simulink model "Guidline_Fuel_Filter_Model"  (R2019a)
settings: Solver=FixedStepDiscrete  StartTime=0.0  StopTime=50  FixedStep=0.01  RelTol=1e-3
undefined symbols (not defined in the file or in its folder): Constant_0, Constant_1, Constant_100, Constant_5, Constant_50, Error_code_101, Error_code_102, resistance_constant
libraries: simulink x2
settings Model: DataDictionary=Fuel_filter_1.sldd  OrderedModelArguments=off  Creator=Akshay  LastModifiedBy=Akshay
settings OptimizationCC: DefaultParameterBehavior=Inlined  UseDivisionForNetSlopeComputation=UseDivisionForReciprocalsOfIntegersOnly  EnhancedBackFolding=on  PassReuseOutputArgsAs=Individual arguments  OptimizeBlockOrder=speed  DifferentSizesBufferReuse=on  OptimizationCustomize=off
settings DebuggingCC: SignalInfNanChecking=warning  ParameterOverflowMsg=none  ParameterTunabilityLossMsg=error  UniqueDataStoreMsg=warning  AssertControl=DisableAll  StrictBusMsg=ErrorOnBusTreatedAsVector  SFUndirectedBroadcastEventsDiag=error
settings SFSimCC: CompileTimeRecursionLimit=0  EnableRuntimeRecursion=off  MATLABDynamicMemAlloc=off
settings RTWCC: SystemTargetFile=ert.tlc  GenCodeOnly=on  TemplateMakefile=ert_default_tmf  GenerateReport=on  IncludeHyperlinkInReport=on  LaunchReport=on  GenerateTraceInfo=on  GenerateTraceReport=on  GenerateTraceReportSl=on  GenerateTraceReportSf=on  GenerateTraceReportEml=on
settings CodeAppCC: ForceParamTrailComments=on  IgnoreCustomStorageClasses=off  OperatorAnnotations=on  SimulinkDataObjDesc=on  SFDataObjDesc=on  MATLABFcnDesc=on  InsertBlockDesc=on
settings ERTTargetCC: TargetLangStandard=C99 (ISO)  UtilityFuncGeneration=Shared location  GenerateSampleERTMain=on  SupportNonFinite=off  ParenthesesLevel=Maximum  CastingMode=Standards  GenerateSharedConstants=off  InlinedParameterPlacement=NonHierarchical  ERTCustomFileTemplate=example_file_process.tlc  EnableSignedLeftShifts=off  EnableSignedRightShifts=off
settings ConfigComp: CovMetricSettings=dcmwe  DVMaxProcessTime=1000  DVParametersUseConfig=on  DVModelCoverageObjectives=MCDC  DVTestSuiteOptimization=Auto  DVDetectOutOfBounds=on  DVDetectInfNaN=on  DVDetectSubnormal=on  DVDesignMinMaxCheck=on  DVProvingStrategy=ProveWithViolationDetection  DVSaveReport=on  DVReportPDFFormat=on  DVRebuildModelRepresentation=Always

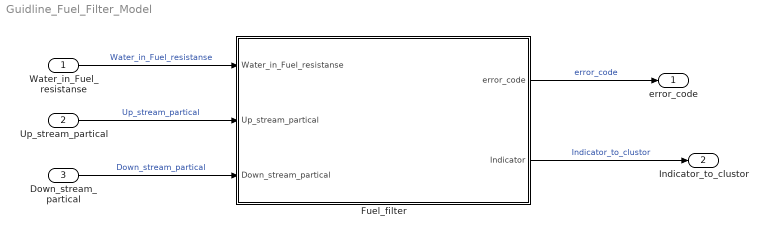
== system Guidline_Fuel_Filter_Model ==
  Water_in_Fuel_resistanse : Inport  OutDataTypeStr=single
  Up_stream_partical : Inport  Port=2  OutDataTypeStr=single
  Down_stream_partical : Inport  Port=3  OutDataTypeStr=single
  Fuel_filter : Subsystem  TreatAsAtomicUnit=on
  error_code : Outport  OutDataTypeStr=single
  Indicator_to_clustor : Outport  Port=2  OutDataTypeStr=boolean
  wires:
  Fuel_filter/1(error_code) -> error_code/1  "error_code"
  Fuel_filter/2(Indicator) -> Indicator_to_clustor/1  "Indicator_to_clustor"
  Water_in_Fuel_resistanse/1 -> Fuel_filter/1(Water_in_Fuel_resistanse)  "Water_in_Fuel_resistanse"
  Up_stream_partical/1 -> Fuel_filter/2(Up_stream_partical)  "Up_stream_partical"
  Down_stream_partical/1 -> Fuel_filter/3(Down_stream_partical)  "Down_stream_partical"

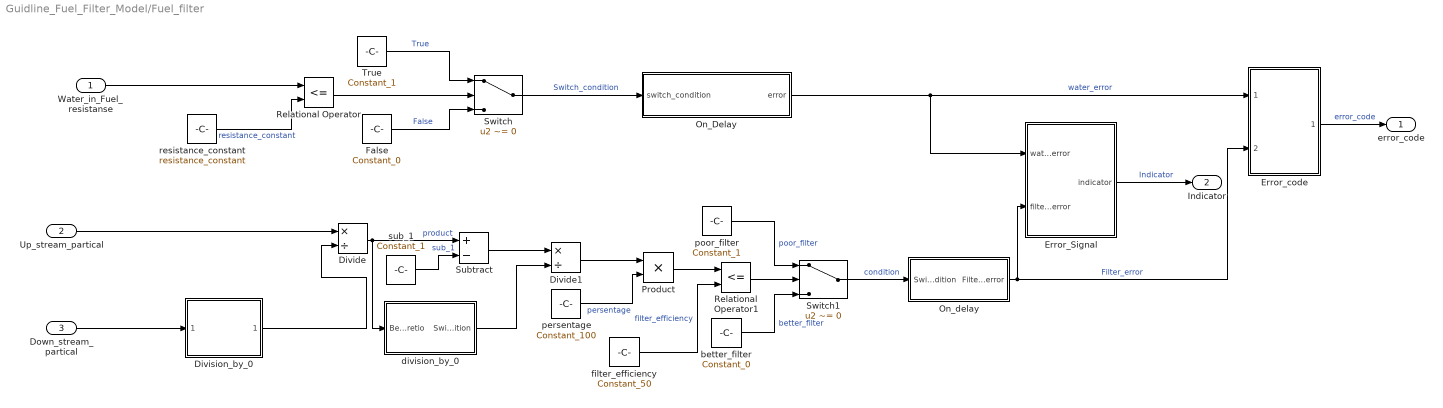
== system Guidline_Fuel_Filter_Model/Fuel_filter ==
  Water_in_Fuel_resistanse : Inport  OutDataTypeStr=single
  Up_stream_partical : Inport  Port=2  OutDataTypeStr=single
  Down_stream_partical : Inport  Port=3  OutDataTypeStr=single
  Divide : Product  Inputs=*/  OutDataTypeStr=single  RndMeth=Ceiling
  Divide1 : Product  Inputs=*/  OutDataTypeStr=single  RndMeth=Ceiling
  Division_by_0 : Subsystem  TreatAsAtomicUnit=on
  Error_Signal : Subsystem  TreatAsAtomicUnit=on
  Error_code : Subsystem  TreatAsAtomicUnit=on
  False : Constant  Value=Constant_0  OutDataTypeStr=single
  On_Delay : Subsystem  TreatAsAtomicUnit=on
  On_delay : Subsystem  TreatAsAtomicUnit=on
  Product : Product  OutDataTypeStr=single  RndMeth=Ceiling
  Relational Operator : RelationalOperator  Operator=<=  OutDataTypeStr=boolean  RndMeth=Simplest
  Relational Operator1 : RelationalOperator  Operator=<=  OutDataTypeStr=boolean  RndMeth=Simplest
  Subtract : Sum  Inputs=+-  AccumDataTypeStr=single  OutDataTypeStr=single  RndMeth=Ceiling
      settings: AttributesFormatString=|
      | AccumDataTypeStr=%<AccumDataTypeStr>
      | RndMeth=%<RndMeth>
  Switch : Switch  Criteria=u2 ~= 0  OutDataTypeStr=single
  Switch1 : Switch  Criteria=u2 ~= 0  OutDataTypeStr=single
  True : Constant  Value=Constant_1  OutDataTypeStr=single
  better_filter : Constant  Value=Constant_0  OutDataTypeStr=single
  division_by_0 : Subsystem  TreatAsAtomicUnit=on
  filter_efficiency : Constant  Value=Constant_50  OutDataTypeStr=single
  persentage : Constant  Value=Constant_100  OutDataTypeStr=single
  poor_filter : Constant  Value=Constant_1  OutDataTypeStr=single
  resistance_constant : Constant  Value=resistance_constant  OutDataTypeStr=single
  "sub_1 " : Constant  Value=Constant_1  OutDataTypeStr=single
  error_code : Outport  OutDataTypeStr=single
  Indicator : Outport  Port=2  OutDataTypeStr=boolean
  wires:
  Water_in_Fuel_resistanse/1 -> Relational Operator/1
  Relational Operator/1 -> Switch/2
  True/1 -> Switch/1  "True"
  False/1 -> Switch/3  "False"
  Up_stream_partical/1 -> Divide/1
  Divide/1 -> Subtract/1, division_by_0/1(Beeta_retio)  "product"
  "sub_1 "/1 -> Subtract/2  "sub_1"
  Subtract/1 -> Divide1/1
  Divide1/1 -> Product/1
  persentage/1 -> Product/2  "persentage"
  Product/1 -> Relational Operator1/1
  Relational Operator1/1 -> Switch1/2
  poor_filter/1 -> Switch1/1  "poor_filter"
  better_filter/1 -> Switch1/3  "better_filter"
  Switch1/1 -> On_delay/1(Switch_condition)  "condition"
  Error_code/1(Error_code) -> error_code/1  "error_code"
  Switch/1 -> On_Delay/1(switch_condition)  "Switch_condition"
  Error_Signal/1(indicator) -> Indicator/1  "Indicator"
  resistance_constant/1 -> Relational Operator/2  "resistance_constant"
  filter_efficiency/1 -> Relational Operator1/2  "filter_efficiency"
  On_Delay/1(error) -> Error_Signal/1(water_error), Error_code/1(water_error)  "water_error"
  On_delay/1(Filter_error) -> Error_code/2(Filter_error), Error_Signal/2(filter_error)  "Filter_error"
  Down_stream_partical/1 -> Division_by_0/1(Down_stream_partical)
  Division_by_0/1(Downstream_partical) -> Divide/2
  division_by_0/1(Switch_condition) -> Divide1/2

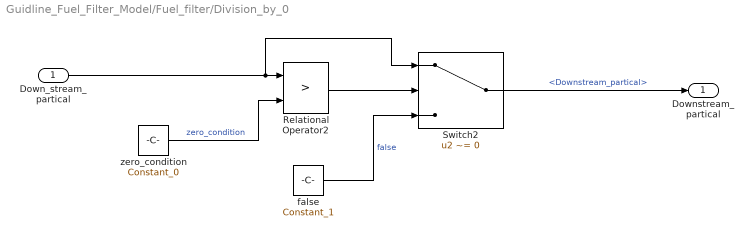
== system Guidline_Fuel_Filter_Model/Fuel_filter/Division_by_0 ==
  Down_stream_partical : Inport  OutDataTypeStr=single
  Relational Operator2 : RelationalOperator  Operator=>  OutDataTypeStr=boolean  RndMeth=Simplest
  Switch2 : Switch  Criteria=u2 ~= 0  OutDataTypeStr=single
  false : Constant  Value=Constant_1  OutDataTypeStr=single
  zero_condition : Constant  Value=Constant_0  OutDataTypeStr=single
  Downstream_partical : Outport  OutDataTypeStr=single
  wires:
  zero_condition/1 -> Relational Operator2/2  "zero_condition"
  Down_stream_partical/1 -> Switch2/1, Relational Operator2/1
  Switch2/1 -> Downstream_partical/1  "<Downstream_partical>"
  false/1 -> Switch2/3  "false"
  Relational Operator2/1 -> Switch2/2

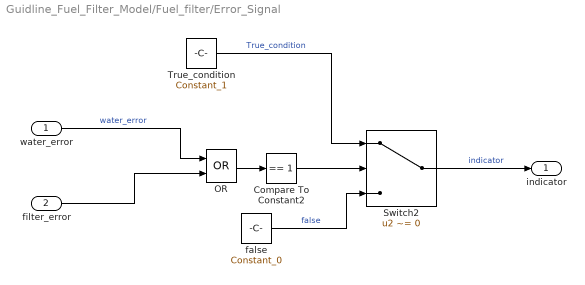
== system Guidline_Fuel_Filter_Model/Fuel_filter/Error_Signal ==
  water_error : Inport  OutDataTypeStr=boolean
  filter_error : Inport  Port=2  OutDataTypeStr=boolean
  Compare To Constant2 : simulink/Logic and Bit Operations/Compare To Constant  relop===  const=1  OutDataTypeStr=boolean
  OR : Logic  Operator=OR  AllPortsSameDT=off  OutDataTypeStr=boolean
  Switch2 : Switch  Criteria=u2 ~= 0  OutDataTypeStr=boolean
  True_condition : Constant  Value=Constant_1  OutDataTypeStr=single
  false : Constant  Value=Constant_0  OutDataTypeStr=single
  indicator : Outport  OutDataTypeStr=boolean
  wires:
  filter_error/1 -> OR/2
  water_error/1 -> OR/1  "water_error"
  Compare To Constant2/1 -> Switch2/2
  True_condition/1 -> Switch2/1  "True_condition"
  OR/1 -> Compare To Constant2/1
  Switch2/1 -> indicator/1  "indicator"
  false/1 -> Switch2/3  "false"

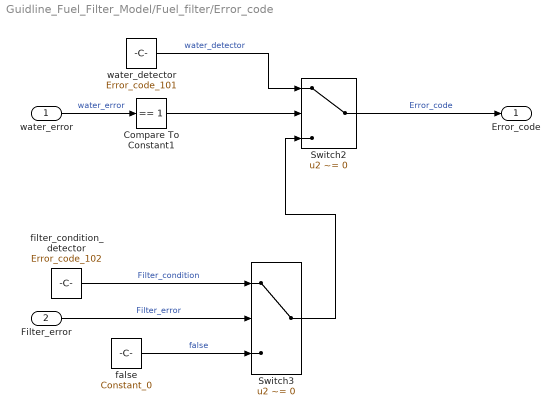
== system Guidline_Fuel_Filter_Model/Fuel_filter/Error_code ==
  water_error : Inport  OutDataTypeStr=boolean
  Filter_error : Inport  Port=2  OutDataTypeStr=boolean
  Compare To Constant1 : simulink/Logic and Bit Operations/Compare To Constant  relop===  const=1  OutDataTypeStr=boolean
  Switch2 : Switch  Criteria=u2 ~= 0  OutDataTypeStr=single
  Switch3 : Switch  Criteria=u2 ~= 0  OutDataTypeStr=single
  false : Constant  Value=Constant_0  OutDataTypeStr=single
  filter_condition_detector : Constant  Value=Error_code_102  OutDataTypeStr=single
  water_detector : Constant  Value=Error_code_101  OutDataTypeStr=int8
  Error_code : Outport  OutDataTypeStr=single
  wires:
  Switch3/1 -> Switch2/3
  filter_condition_detector/1 -> Switch3/1  "Filter_condition"
  Switch2/1 -> Error_code/1  "Error_code"
  water_error/1 -> Compare To Constant1/1  "water_error"
  water_detector/1 -> Switch2/1  "water_detector"
  Filter_error/1 -> Switch3/2  "Filter_error"
  false/1 -> Switch3/3  "false"
  Compare To Constant1/1 -> Switch2/2

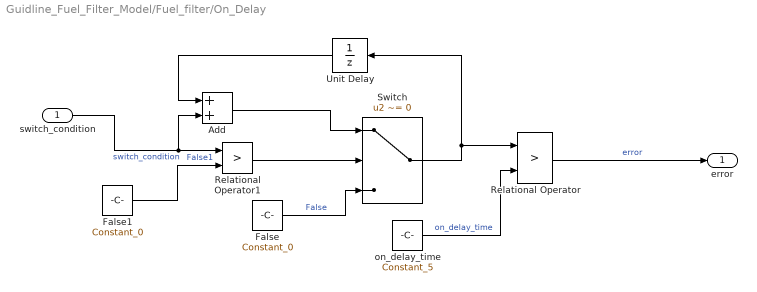
== system Guidline_Fuel_Filter_Model/Fuel_filter/On_Delay ==
  switch_condition : Inport  OutDataTypeStr=single
  Add : Sum  AccumDataTypeStr=single  OutDataTypeStr=single
      settings: AttributesFormatString=AccumDataTypeStr=%<AccumDataTypeStr>
  False : Constant  Value=Constant_0  OutDataTypeStr=single
  False1 : Constant  Value=Constant_0  OutDataTypeStr=single
  Relational Operator : RelationalOperator  Operator=>  OutDataTypeStr=boolean  RndMeth=Simplest
  Relational Operator1 : RelationalOperator  Operator=>  OutDataTypeStr=boolean  RndMeth=Simplest
  Switch : Switch  Criteria=u2 ~= 0  OutDataTypeStr=single
  Unit Delay : UnitDelay  SampleTime=-1  HasFrameUpgradeWarning=on
  on_delay_time : Constant  Value=Constant_5  OutDataTypeStr=single
  error : Outport  OutDataTypeStr=boolean
  wires:
  Switch/1 -> Unit Delay/1, Relational Operator/1
  switch_condition/1 -> Relational Operator1/1, Add/2  "switch_condition"
  False/1 -> Switch/3  "False"
  Add/1 -> Switch/1
  Unit Delay/1 -> Add/1
  Relational Operator/1 -> error/1  "error"
  on_delay_time/1 -> Relational Operator/2  "on_delay_time"
  Relational Operator1/1 -> Switch/2
  False1/1 -> Relational Operator1/2  "False1"

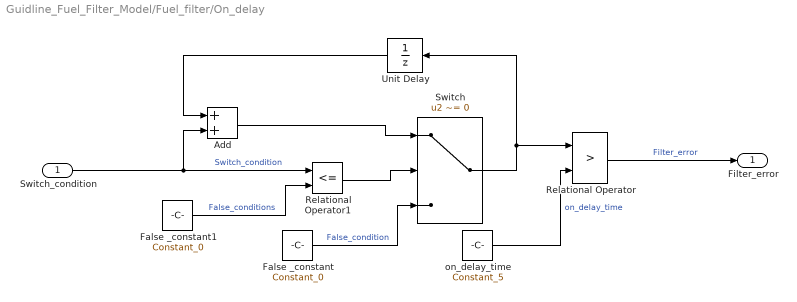
== system Guidline_Fuel_Filter_Model/Fuel_filter/On_delay ==
  Switch_condition : Inport  OutDataTypeStr=single
  Add : Sum  AccumDataTypeStr=single  OutDataTypeStr=single
      settings: AttributesFormatString=AccumDataTypeStr=%<AccumDataTypeStr>
  False _constant : Constant  Value=Constant_0  OutDataTypeStr=boolean
  False _constant1 : Constant  Value=Constant_0  OutDataTypeStr=boolean
  Relational Operator : RelationalOperator  Operator=>  OutDataTypeStr=boolean  RndMeth=Simplest
  Relational Operator1 : RelationalOperator  Operator=<=  OutDataTypeStr=boolean  RndMeth=Simplest
  Switch : Switch  Criteria=u2 ~= 0  OutDataTypeStr=single
  Unit Delay : UnitDelay  SampleTime=-1  HasFrameUpgradeWarning=on
  on_delay_time : Constant  Value=Constant_5  OutDataTypeStr=single
  Filter_error : Outport  OutDataTypeStr=boolean
  wires:
  on_delay_time/1 -> Relational Operator/2  "on_delay_time"
  Relational Operator/1 -> Filter_error/1  "Filter_error"
  Unit Delay/1 -> Add/1
  Add/1 -> Switch/1
  False _constant/1 -> Switch/3  "False_condition"
  Switch_condition/1 -> Relational Operator1/1, Add/2  "Switch_condition"
  Switch/1 -> Relational Operator/1, Unit Delay/1
  Relational Operator1/1 -> Switch/2
  False _constant1/1 -> Relational Operator1/2  "False_conditions"

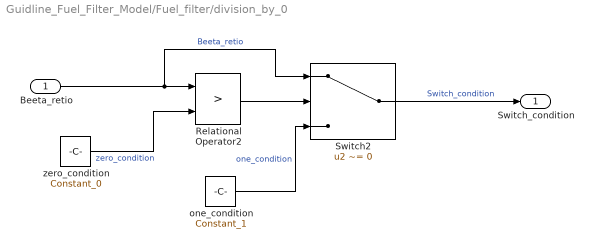
== system Guidline_Fuel_Filter_Model/Fuel_filter/division_by_0 ==
  Beeta_retio : Inport  OutDataTypeStr=single
  Relational Operator2 : RelationalOperator  Operator=>  OutDataTypeStr=boolean  RndMeth=Simplest
  Switch2 : Switch  Criteria=u2 ~= 0  OutDataTypeStr=single
  one_condition : Constant  Value=Constant_1  OutDataTypeStr=single
  zero_condition : Constant  Value=Constant_0  OutDataTypeStr=single
  Switch_condition : Outport  OutDataTypeStr=single
  wires:
  Relational Operator2/1 -> Switch2/2
  one_condition/1 -> Switch2/3  "one_condition"
  Switch2/1 -> Switch_condition/1  "Switch_condition"
  Beeta_retio/1 -> Relational Operator2/1, Switch2/1  "Beeta_retio"
  zero_condition/1 -> Relational Operator2/2  "zero_condition"
